simulink library "plant1turb_cl"  (R2020a)
settings: Solver=VariableStepAuto  StartTime=0.0  StopTime=10.0  RelTol=1e-3
undefined symbols (not defined in the file or in its folder): initializeBussesFromBlock
libraries: dspstat3 x1, groundStation_cl x1, tethers_cl x1, vehicle_cl x1, winch_cl x1
settings Model: Creator=mcobb  LastModifiedBy=andre
settings DataIOCC: ReturnWorkspaceOutputs=off
settings DebuggingCC: ArithmeticOperatorsInVariantConditions=warning
settings SFSimCC: CustomCodeUndefinedFunction=UseInterfaceOnly

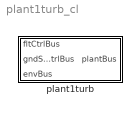
== system plant1turb_cl ==
  plant1turb : Subsystem  LoadFcn=initializeBussesFromBlock(gcb)  InitFcn=initializeBussesFromBlock(gcb)  StartFcn=initializeBussesFromBlock(gcb)  VariantControl=VSS_plant_modularPlant

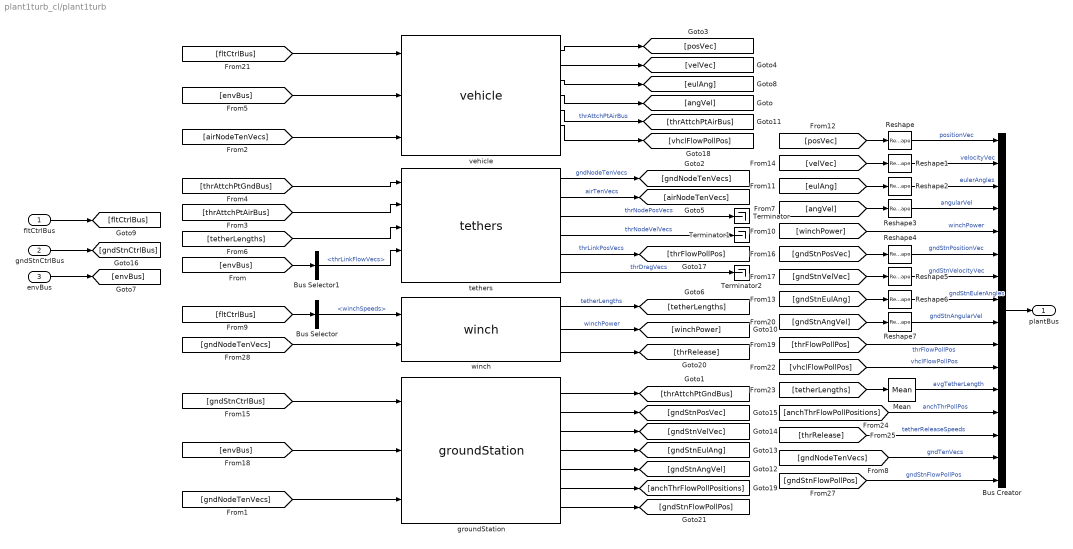
== system plant1turb_cl/plant1turb ==
  fltCtrlBus : Inport  OutDataTypeStr=Bus: fltCtrlBus
  gndStnCtrlBus : Inport  Port=2  OutDataTypeStr=Bus: gndStnCtrlBus
  envBus : Inport  Port=3  OutDataTypeStr=Bus: envBus
  Bus Creator : BusCreator  Inputs=16  OutDataTypeStr=Bus: plantBus  NonVirtualBus=on
  Bus Selector : BusSelector  OutputSignals=winchSpeeds
  Bus Selector1 : BusSelector  OutputSignals=thrLinkFlowVecs
  Mean : dspstat3/Mean  run=off  InputProcessing=Columns as channels (frame based)  reset_popup=None  directionMode=Each column  dimension=1  roiEnable=off  roiType=Rectangles  roiPortion=Entire ROI  roiOutput=Individual statistics for each ROI  roiFlag=off  roundingMode=Floor  overflowMode=off  outputDataTypeStr=Inherit: Same as accumulator  outputMin=[]  outputMax=[]  outputLastDataTypeStr=Inherit: Same as accumulator
  Reshape{,1..7} (8 alike) : Reshape  OutputDimensionality=Column vector (2-D)
  Terminator : Terminator
  Terminator1 : Terminator
  Terminator2 : Terminator
  groundStation : groundStation_cl/groundStation  numNodes=2
  tethers : tethers_cl/tethers  SystemSampleTime=-1  Latency=0  AutoFrameSizeCalculation=off
  vehicle : vehicle_cl/vehicle  SystemSampleTime=-1  Latency=0  AutoFrameSizeCalculation=off
  winch : winch_cl/winch  SystemSampleTime=-1  Latency=0  AutoFrameSizeCalculation=off
  plantBus : Outport  OutDataTypeStr=Bus: plantBus  VectorParamsAs1DForOutWhenUnconnected=off
  wires:
  envBus/1 -> [envBus]
  fltCtrlBus/1 -> [fltCtrlBus]
  Bus Creator/1 -> plantBus/1
  Reshape/1 -> Bus Creator/1  "positionVec"
  Reshape2/1 -> Bus Creator/3  "eulerAngles"
  Reshape1/1 -> Bus Creator/2  "velocityVec"
  winch/1 -> [tetherLengths]  "tetherLengths"
  [posVec] -> Reshape/1
  [velVec] -> Reshape1/1
  [eulAng] -> Reshape2/1
  vehicle/3 -> [eulAng]
  vehicle/1 -> [posVec]
  vehicle/5 -> [thrAttchPtAirBus]  "thrAttchPtAirBus"
  vehicle/2 -> [velVec]
  vehicle/4 -> [angVel]
  [envBus] -> Bus Selector1/1
  groundStation/1 -> [thrAttchPtGndBus]
  tethers/1 -> [gndNodeTenVecs]  "gndNodeTenVecs"
  tethers/2 -> [airNodeTenVecs]  "airTenVecs"
  tethers/3 -> Terminator/1  "thrNodePosVecs"
  [gndNodeTenVecs] -> groundStation/3
  [airNodeTenVecs] -> vehicle/3
  [thrAttchPtAirBus] -> tethers/2
  [thrAttchPtGndBus] -> tethers/1
  [tetherLengths] -> tethers/3
  [envBus] -> groundStation/2
  [gndStnCtrlBus] -> groundStation/1
  [fltCtrlBus] -> vehicle/1
  [envBus] -> vehicle/2
  [fltCtrlBus] -> Bus Selector/1
  [angVel] -> Reshape3/1
  Reshape3/1 -> Bus Creator/4  "angularVel"
  winch/2 -> [winchPower]  "winchPower"
  [winchPower] -> Bus Creator/5  "winchPower"
  [gndStnAngVel] -> Reshape7/1
  [gndStnEulAng] -> Reshape6/1
  [gndStnVelVec] -> Reshape5/1
  [gndStnPosVec] -> Reshape4/1
  Reshape4/1 -> Bus Creator/6  "gndStnPositionVec"
  Reshape5/1 -> Bus Creator/7  "gndStnVelocityVec"
  Reshape6/1 -> Bus Creator/8  "gndStnEulerAngles"
  Reshape7/1 -> Bus Creator/9  "gndStnAngularVel"
  groundStation/2 -> [gndStnPosVec]
  groundStation/3 -> [gndStnVelVec]
  groundStation/4 -> [gndStnEulAng]
  groundStation/5 -> [gndStnAngVel]
  gndStnCtrlBus/1 -> [gndStnCtrlBus]
  Bus Selector/1 -> winch/1  "<winchSpeeds>"
  winch/3 -> [thrRelease]
  tethers/4 -> Terminator1/1  "thrNodeVelVecs"
  [thrFlowPollPos] -> Bus Creator/10  "thrFlowPollPos"
  vehicle/6 -> [vhclFlowPollPos]
  [vhclFlowPollPos] -> Bus Creator/11  "vhclFlowPollPos"
  Bus Selector1/1 -> tethers/4  "<thrLinkFlowVecs>"
  [tetherLengths] -> Mean/1
  Mean/1 -> Bus Creator/12  "avgTetherLength"
  groundStation/6 -> [anchThrFlowPollPositions]
  [anchThrFlowPollPositions] -> Bus Creator/13  "anchThrPollPos"
  [thrRelease] -> Bus Creator/14  "tetherReleaseSpeeds"
  [gndNodeTenVecs] -> Bus Creator/15  "gndTenVecs"
  groundStation/7 -> [gndStnFlowPollPos]
  [gndStnFlowPollPos] -> Bus Creator/16  "gndStnFlowPollPos"
  tethers/5 -> [thrFlowPollPos]  "thrLinkPosVecs"
  [gndNodeTenVecs] -> winch/2
  tethers/6 -> Terminator2/1  "thrDragVecs"
